simulink model "Week1_Problem3"  (R2019b)
settings: Solver=VariableStepAuto  StartTime=0.0  StopTime=10.0  RelTol=1e-3
model workspace (MAT data in the model file):
  a1 = 0.01584
  b0 = 0.5792
  b1 = -0.5792
settings Model: Creator=Shreyas  LastModifiedBy=Shreyas

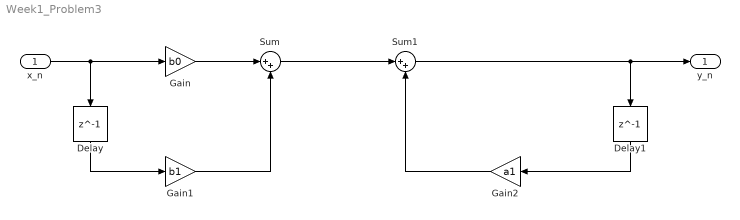
== system Week1_Problem3 ==
  x_n : Inport
  Delay : Delay  DelayLength=1
  Delay1 : Delay  DelayLength=1
  Gain : Gain  Gain=b0
  Gain1 : Gain  Gain=b1
  Gain2 : Gain  Gain=a1
  Sum : Sum  Inputs=|++
  Sum1 : Sum  Inputs=|++
  y_n : Outport
  wires:
  Delay/1 -> Gain1/1
  x_n/1 -> Gain/1, Delay/1
  Gain2/1 -> Sum1/2
  Sum/1 -> Sum1/1
  Gain1/1 -> Sum/2
  Delay1/1 -> Gain2/1
  Gain/1 -> Sum/1
  Sum1/1 -> Delay1/1, y_n/1
